simulink model "Udan_SOC"  (R2017b)
settings: Solver=FixedStepAuto  StartTime=0.0  StopTime=1000  FixedStep=0.1  RelTol=1e-3
values from neighbouring files (symbols this model uses):
  DenominatorOfIntegratorFactor = 100.0    [SOC_Stateflow.sldd]
  SOC_CalcSohLKT = 1.0    [SOC_Stateflow.sldd]
  SOC_CalcSOHTempLimit = 70.0    [SOC_Stateflow.sldd]
  SOC_CapPerCycle = 100.0    [SOC_Stateflow.sldd]
  SOC_CapTemp_HLimit = 200.0    [SOC_Stateflow.sldd]
  SOC_CapTemp_LLimit = 0.0    [SOC_Stateflow.sldd]
  Soc_ConfigInfo = 0    [SOC_Stateflow.sldd]
  SOC_DchgEndCalib = 0.0    [SOC_Stateflow.sldd]
  SOC_DiffVoltMin = 10.0    [SOC_Stateflow.sldd]
  SOC_DSOCJumpMax = 500.0    [SOC_Stateflow.sldd]
  SOC_EfficientHighLimit = 250.0    [SOC_Stateflow.sldd]
  SOC_EfficientLowLimit = 40.0    [SOC_Stateflow.sldd]
  SOC_EmptyAus = 0.0    [SOC_Stateflow.sldd]
  SOC_EnableOcv = 1.0    [SOC_Stateflow.sldd]
  SOC_END_CALIB_STATE : value not decoded    [SOC_Stateflow.sldd]
  SOC_HighRealSoc = 95.0    [SOC_Stateflow.sldd]
  SOC_LKTSohCycles = 0.0 1.0 10.0 20.0 30.0 40.0 50.0 60.0 70.0 80.0 90.0 100.0 110.0 120.0 130.0 140.0 150.0 160.0 170.0 180.0 190.0 200.0 210.0 220.0 230.0 240.0 250.0 260.0 270.0 280.0 290.0 300.0 310.0 320.0 330.0 340.0 350.0 360.0 370.0 380.0 390.0 400.0 410.0 420.0 430.0 440.0 450.0 460.0 470.0 480.0 490.0 500.0 510.0 520.0 530.0 540.0 550.0 560.0 570.0 580.0 590.0 600.0 610.0 620.0 630.0 640.0 650.0 660.0 670.0    [SOC_Stateflow.sldd]
  SOC_LKTSohTable = 1000.0 991.0 989.0 992.0 993.0 995.0 994.0 993.0 1000.0 997.0 1002.0 1000.0 992.0 1000.0 989.0 992.0 989.0 994.0 989.0 993.0 994.0 994.0 994.0 993.0 991.0 991.0 992.0 993.0 991.0 985.0 985.0 985.0 979.0 975.0 978.0 984.0 982.0 974.0 975.0 972.0 972.0 975.0 977.0 977.0 974.0 971.0 973.0 971.0 966.0 968.0 965.0 959.0 957.0 956.0 957.0 954.0 955.0 951.0 954.0 951.0 942.0 942.0 940.0 942.0 947.0 949.0    [SOC_Stateflow.sldd]
  SOC_LowRealSoc = 5.0    [SOC_Stateflow.sldd]
  SOC_NominalCap_AmS = 576000000.0    [SOC_Stateflow.sldd]
  SOC_NominalVol = 4000.0    [SOC_Stateflow.sldd]
  SOC_OCVTemp_HLimit = 106.0    [SOC_Stateflow.sldd]
  SOC_OCVTemp_LLimit = 29.0    [SOC_Stateflow.sldd]
  SOC_ShortCalibDSoc = 1.0    [SOC_Stateflow.sldd]
  SOC_SOCResolution = 10000.0    [SOC_Stateflow.sldd]
  SOC_SohCalcCapPercent = 8.0    [SOC_Stateflow.sldd]
  SOC_SohCalcHighLimit = 60.0    [SOC_Stateflow.sldd]
  SOC_SohCalcLowLimit = 10.0    [SOC_Stateflow.sldd]
  SOC_SohCalcMidLimit = 30.0    [SOC_Stateflow.sldd]
  SOC_SOHResolution = 1000.0    [SOC_Stateflow.sldd]
  SOC_State = <binary blob, 1163 chars, not shown>    [SOC_Stateflow.sldd]
  SOC_TempCap_CapBuffer : value not decoded    [SOC_Stateflow.sldd]
  SOC_TempCap_TempBuffer : value not decoded    [SOC_Stateflow.sldd]
  SocOcvCalib_ConfigInfo = 0.0    [SOC_Stateflow.sldd]
  SocOcvCalib_SocBuffer1 : value not decoded    [SOC_Stateflow.sldd]
  SocOcvCalib_TempBuffer : value not decoded    [SOC_Stateflow.sldd]
  SocOcvCalib_VoltageBuffer1 = 3300.0 3303.0 3305.0 3307.0 3310.0 3311.0 3313.0 3314.0 3316.0 3317.0 3319.0 3320.0 3322.0 3323.0 3325.0 3322.0 3323.0 3325.0 3310.0 3313.0 3315.0 3317.0 3320.0 3321.0 3323.0 3324.0 3326.0 3327.0 3329.0 3330.0 3332.0 3333.0 3335.0 3332.0 3333.0 3335.0 3320.0 3323.0 3325.0 3327.0 3330.0 3331.0 3333.0 3334.0 3336.0 3337.0 3339.0 3340.0 3342.0 3343.0 3345.0 3342.0 3343.0 3345.0 3330.0 3333.0 3335.0 3    [SOC_Stateflow.sldd]
  SOHCalibCycle = 10.0    [SOC_Stateflow.sldd]
undefined symbols (not defined in the file or in its folder): DatetimeM_GetReturnType, ParameterM_EeepParaIndexType, Soc_CumuLativeTypeType, SOC_EgthTempChgValue, Soc_EnergyBuffer, SOC_FithTempChgValue, SOC_FstSlowTempChgValue, SOC_FstTempChgValue, SOC_FthTempChgValue, SOC_MaxCap_AmS, SOC_SethTempChgValue, SOC_SixTempChgValue, SOC_SndSlowTempChgValue, SOC_SndTempChgValue, SOC_TrdSlowTempChgValue, SOC_TrdTempChgValue, SocDiagCalib_NoCalibReasonType
libraries: simulink x138, hdlsllib x24, dspindex x4
(part 2 of 10)

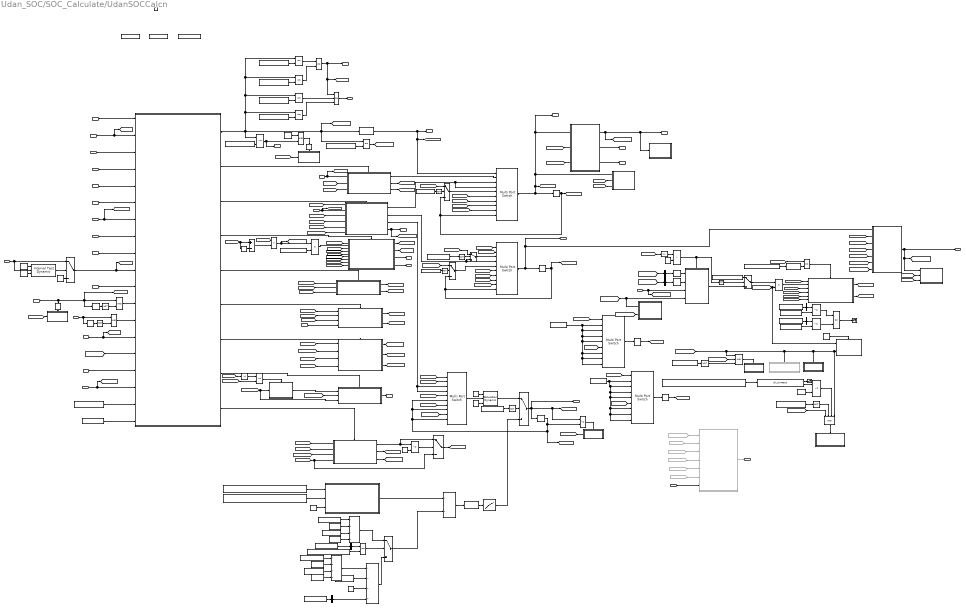
== system Udan_SOC/SOC_Calculate/UdanSOCCalcn ==
  note: 充电连接或者断开将未进行末端校正的累积安时数清0
  RtcTimeIsOk : Inport
  RtcTime : Inport  Port=2
  IsCharging : Inport  Port=3
  BmuStateIsOk : Inport  Port=4
  LongBatOffTimeOk : Inport  Port=5
  BatOffTimeOk : Inport  Port=6
  SohTimeOk : Inport  Port=7
  CalibCurrentMax : Inport  Port=8
  CalibCheckCycle : Inport  Port=9
  CalibWriteCycle : Inport  Port=10
  powerOnDelay : Inport  Port=11
  Current : Inport  Port=12
  LastOcvTime : Inport  Port=13
  FullChgFns : Inport  Port=14
  EmptyDchgFlag : Inport  Port=15
  EmptyValue : Inport  Port=16
  TimeStamps : Inport  Port=17
  CellLowTemp : Inport  Port=18
  UCell : Inport  Port=19
  SocCalibFlag : Inport  Port=20  OutDataTypeStr=uint8  PortDimensions=[1]
  BatHighTemp : Inport  Port=21
  Enable : EnablePort
  1-D Lookup Table : Lookup_n-D  NumberOfTableDimensions=1  BreakpointsForDimension1=SOC_LKTSohCycles  Table=SOC_LKTSohTable  ExtrapMethod=Clip  InternalRulePriority=Speed  OutDataTypeStr=uint16  RndMeth=Simplest
  Abs : Abs
  Abs1 : Abs
  Bus Selector : BusSelector  OutputSignals=soc
  Bus Selector1 : BusSelector  OutputSignals=soc
  Bus Selector2 : BusSelector  OutputSignals=DchgCumuInfo.resoltion
  Bus Selector4 : BusSelector  OutputSignals=DchgCumuInfo.type
  Bus Selector7 : BusSelector  OutputSignals=ChgCumuInfo.type
  Bus Selector8 : BusSelector  OutputSignals=DchgCumuInfo.type
  CalcChgSOH : Subsystem  TreatAsAtomicUnit=on
  CalcDchgSOH : Subsystem  TreatAsAtomicUnit=on
  CalcSocEffiient : Subsystem
  CalclnCore : Stateflow chart  TreatAsAtomicUnit=on
  CalcnLeftChargeTime : Subsystem  Commented=on
  CalcnSOC : Subsystem
  CalcnSOC1 : Subsystem
  CalibEmptySOC : Subsystem  TreatAsAtomicUnit=on
  CalibFullSOC : Subsystem  TreatAsAtomicUnit=on
  CapAdder1 : Subsystem
  CapAdder2 : Subsystem
  ClearLeftCapWOCalib : Subsystem  Commented=on
  ClearLeftCapWOCalib2 : Subsystem  TreatAsAtomicUnit=on
  ClearSOHCalcFlag : Subsystem  TreatAsAtomicUnit=on
  Constant : Constant  Value=0  OutDataTypeStr=uint8
  Constant1 : Constant  Value=DenominatorOfIntegratorFactor  OutDataTypeStr=uint16
  Constant10 : Constant  Value=600  OutDataTypeStr=uint16
  Constant11 : Constant  Value=0  OutDataTypeStr=uint32
  Constant12 : Constant  Value=0  OutDataTypeStr=int16
  Constant{13..14,25,27} (4 alike) : Constant  Value=Soc_ConfigInfo  OutDataTypeStr=Bus: Soc_ConfigInfoType
  Constant15 : Constant  Value=0  OutDataTypeStr=boolean
  Constant16 : Constant  Value=SOC_NominalCap_AmS
  Constant17 : Constant  Value=3600000  OutDataTypeStr=uint32
  Constant18 : Constant  Value=SOC_CalcSohLKT
  Constant19 : Constant  Value=SOC_CalcSohLKT
  Constant2 : Constant  Value=0
  Constant20 : Constant  Value=SOC_ShortCalibDSoc
  Constant21 : Constant  Value=SOC_CalcSohLKT
  Constant22 : Constant  Value=SOC_CapPerCycle  OutDataTypeStr=uint8
  Constant23 : Constant  Value=100  OutDataTypeStr=uint8
  Constant24 : Constant  OutDataTypeStr=boolean
  Constant26 : Constant  Value=10  OutDataTypeStr=uint8
  Constant28 : Constant  Value=SOC_NominalVol
  Constant29 : Constant  Value=SOC_NominalCap_AmS
  Constant3 : Constant  Value=65535  OutDataTypeStr=uint16
  Constant30 : Constant  Value=3600000  OutDataTypeStr=uint32
  Constant31 : Constant  Value=SOC_CapPerCycle  OutDataTypeStr=uint8
  Constant32 : Constant  Value=100  OutDataTypeStr=uint8
  Constant34 : Constant  Value=SOC_EnableOcv
  Constant4 : Constant  Value=SOC_EmptyAus
  Constant5 : Constant  Value=SOC_EmptyAus
  Constant6 : Constant  Value=20000  OutDataTypeStr=int16
  Constant7 : Constant  Value=-20000  OutDataTypeStr=int16
  Constant8 : Constant  Value=DenominatorOfIntegratorFactor  OutDataTypeStr=uint16
  Constant9 : Constant  Value=1100  OutDataTypeStr=uint16
  DLeftCap : MultiPortSwitch  DataPortOrder=Zero-based contiguous  Inputs=9  DataPortIndices={SOC_STATE_INIT,SOC_STATE_OCV,SOC_STATE_OCV_LONG,SOC_STATE_INTEGRATE,SOC_STATE_FULL}  OutDataTypeStr=uint32
  DLeftCap1 : MultiPortSwitch  DataPortOrder=Zero-based contiguous  Inputs=8  DataPortIndices={SOC_STATE_INIT,SOC_STATE_OCV,SOC_STATE_OCV_LONG,SOC_STATE_INTEGRATE,SOC_STATE_FULL}
  DLeftCap2 : MultiPortSwitch  DataPortOrder=Zero-based contiguous  Inputs=8  DataPortIndices={SOC_STATE_INIT,SOC_STATE_OCV,SOC_STATE_OCV_LONG,SOC_STATE_INTEGRATE,SOC_STATE_FULL}
  Data Store Memory1 : DataStoreMemory  DataStoreName=LargeCurrentFlag  ReadBeforeWriteMsg=warning  WriteAfterWriteMsg=warning  WriteAfterReadMsg=warning  ShowAdditionalParam=off  OutDataTypeStr=boolean
  Data Store Memory2 : DataStoreMemory  DataStoreName=FullFnshFlag  ReadBeforeWriteMsg=warning  WriteAfterWriteMsg=warning  WriteAfterReadMsg=warning  ShowAdditionalParam=off  OutDataTypeStr=boolean
  Data Store Memory4 : DataStoreMemory  DataStoreName=ChgClearWOCalibFlag  ReadBeforeWriteMsg=warning  WriteAfterWriteMsg=warning  WriteAfterReadMsg=warning  ShowAdditionalParam=off  OutDataTypeStr=boolean
  Data Store Read : DataStoreRead  DataStoreName=ChgClearWOCalibFlag
  Data Store Read1 : DataStoreRead  DataStoreName=LargeCurrentFlag
  Data Store Read2 : DataStoreRead  DataStoreName=FullFnshFlag
  Data Type Conversion : DataTypeConversion  OutDataTypeStr=uint8
  Data Type Conversion1 : DataTypeConversion  OutDataTypeStr=uint8
  Data Type Conversion2 : DataTypeConversion
  DchgPower1 : simulink/Sources/Enumerated Constant  OutDataTypeStr=Enum: ParameterM_EeepParaIndexType  Value=ParameterM_EeepParaIndexType.PARAMETERM_EEEP_CUMULATIVE_DCHG_CAP_L_INDEX  SampleTime=inf
      settings: SourceProductName=Simulink
  DchgPower2 : simulink/Sources/Enumerated Constant  OutDataTypeStr=Enum: ParameterM_EeepParaIndexType  Value=ParameterM_EeepParaIndexType.PARAMETERM_EEEP_SOH_Full_INDEX  SampleTime=inf
      settings: SourceProductName=Simulink
  DchgPower3 : simulink/Sources/Enumerated Constant  OutDataTypeStr=Enum: ParameterM_EeepParaIndexType  Value=ParameterM_EeepParaIndexType.PARAMETERM_EEEP_CUMULATIVE_DCHG_CAP_H_INDEX  SampleTime=inf
      settings: SourceProductName=Simulink
  Delay{,1..3,5..11} (11 alike) : Delay  DelayLength=1  InitialCondition=0
  Delay4 : Delay  InitialCondition=0
  Divide : Product  Inputs=*/*/  OutDataTypeStr=uint32
  Divide1 : Product  Inputs=*/  OutDataTypeStr=uint32  RndMeth=Round
  Divide3 : Product  Inputs=**  OutDataTypeStr=int32
  Divide4 : Product  Inputs=**  OutDataTypeStr=int32
  Divide6 : Product  Inputs=*/*/  OutDataTypeStr=uint32
  Divide7 : Product  Inputs=**//  OutDataTypeStr=uint32  RndMeth=Round
  Enabled Subsystem : Subsystem  TreatAsAtomicUnit=on
  Enumerated Constant : simulink/Sources/Enumerated Constant  OutDataTypeStr=Enum: SOC_State  Value=SOC_State.SOC_STATE_INTEGRATE  SampleTime=inf
      settings: SourceProductName=Simulink
  Enumerated Constant1 : simulink/Sources/Enumerated Constant  OutDataTypeStr=Enum: Soc_CumuLativeTypeType  Value=Soc_CumuLativeTypeType.Soc_CumuTypeNone  SampleTime=inf
      settings: SourceProductName=Simulink
  Enumerated Constant12 : simulink/Sources/Enumerated Constant  OutDataTypeStr=Enum: SOC_State  Value=SOC_State.SOC_STATE_INTEGRATE  SampleTime=inf
      settings: SourceProductName=Simulink
  Enumerated Constant2 : simulink/Sources/Enumerated Constant  OutDataTypeStr=Enum: Soc_CumuLativeTypeType  Value=Soc_CumuLativeTypeType.Soc_CumuTypeNone  SampleTime=inf
      settings: SourceProductName=Simulink
  Enumerated Constant3 : simulink/Sources/Enumerated Constant  OutDataTypeStr=Enum: SOC_State  Value=SOC_State.SOC_STATE_INIT  SampleTime=inf
      settings: SourceProductName=Simulink
  Enumerated Constant4 : simulink/Sources/Enumerated Constant  OutDataTypeStr=Enum: SOC_State  Value=SOC_State.SOC_STATE_FULL  SampleTime=inf
      settings: SourceProductName=Simulink
  Enumerated Constant5 : simulink/Sources/Enumerated Constant  OutDataTypeStr=Enum: SOC_State  Value=SOC_State.SOC_STATE_EMPTY  SampleTime=inf
      settings: SourceProductName=Simulink
  Enumerated Constant6 : simulink/Sources/Enumerated Constant  OutDataTypeStr=Enum: SOC_State  Value=SOC_State.SOC_STATE_OCV_LONG  SampleTime=inf
      settings: SourceProductName=Simulink
  Enumerated Constant7 : simulink/Sources/Enumerated Constant  OutDataTypeStr=Enum: SOC_State  Value=SOC_State.SOC_STATE_OCV  SampleTime=inf
      settings: SourceProductName=Simulink
  Enumerated Constant8 : simulink/Sources/Enumerated Constant  OutDataTypeStr=Enum: Soc_CumuLativeTypeType  Value=Soc_CumuLativeTypeType.Soc_CumuTypeCap  SampleTime=inf
      settings: SourceProductName=Simulink
  From74 : From  Commented=on  GotoTag=LastDCapWODelay
  From75 : From  Commented=on  GotoTag=CellTemp
  From77 : From  Commented=on  GotoTag=CurrentSOH
  From78 : From  Commented=on  GotoTag=IsCharging
  From84 : From  Commented=on  GotoTag=TimeStamps
  From92 : From  Commented=on  GotoTag=Current
  Function-Call Subsystem : Subsystem  TreatAsAtomicUnit=on
  Function-Call Subsystem4 : Subsystem  TreatAsAtomicUnit=on
  Interval Test Dynamic : simulink/Logic and Bit Operations/Interval Test Dynamic  IntervalClosedRight=on  IntervalClosedLeft=on  OutDataTypeStr=boolean
      settings: SourceProductName=Simulink  SourceProductBaseCode=SL
  LKTSOC : Subsystem  TreatAsAtomicUnit=on
  LeftCap : MultiPortSwitch  DataPortOrder=Zero-based contiguous  Inputs=9  DataPortIndices={SOC_STATE_INIT,SOC_STATE_OCV,SOC_STATE_OCV_LONG,SOC_STATE_INTEGRATE,SOC_STATE_FULL}  OutDataTypeStr=uint32
  Logical Operator : Logic  Inputs=4  AllPortsSameDT=off  OutDataTypeStr=boolean
  Logical Operator{1,3,8,12..16} (8 alike) : Logic  Operator=NOT  AllPortsSameDT=off  OutDataTypeStr=boolean
  Logical Operator10 : Logic  Operator=OR  AllPortsSameDT=off  OutDataTypeStr=boolean
  Logical Operator11 : Logic  AllPortsSameDT=off  OutDataTypeStr=boolean
  Logical Operator2 : Logic  AllPortsSameDT=off  OutDataTypeStr=boolean
  Logical Operator4 : Logic  Inputs=3  AllPortsSameDT=off  OutDataTypeStr=boolean
  Logical Operator5 : Logic  Operator=OR  AllPortsSameDT=off  OutDataTypeStr=boolean
  Logical Operator6 : Logic  Operator=NOT  Inputs=3  AllPortsSameDT=off  OutDataTypeStr=boolean
  Logical Operator7 : Logic  Operator=OR  Inputs=3  AllPortsSameDT=off  OutDataTypeStr=boolean
  Logical Operator9 : Logic  AllPortsSameDT=off  OutDataTypeStr=boolean
  Multiport Switch1 : MultiPortSwitch  DataPortOrder=Zero-based contiguous  Inputs=9  DataPortIndices={SOC_STATE_INIT,SOC_STATE_OCV,SOC_STATE_OCV_LONG,SOC_STATE_INTEGRATE,SOC_STATE_FULL}
  Product : Product  OutDataTypeStr=int32
  Relational Operator{,7..8,10..12,15} (7 alike) : RelationalOperator  Operator===  OutDataTypeStr=boolean  RndMeth=Simplest
  Relational Operator{1..6} (6 alike) : RelationalOperator  Operator=~=  OutDataTypeStr=boolean  RndMeth=Simplest
  Relational Operator13 : RelationalOperator  OutDataTypeStr=boolean  RndMeth=Simplest
  Relational Operator9 : RelationalOperator  Operator=>  OutDataTypeStr=boolean  RndMeth=Simplest
  S-Function2 : S-Function  FunctionName=sfn_NVMRead  SFunctionDeploymentMode=off  EnableBusSupport=off
  Saturation Dynamic : simulink/Discontinuities/Saturation Dynamic  OutMin=[]  OutMax=[]  OutDataTypeStr=Inherit: Same as second input  OutDataType=fixdt(1, 16)  OutScaling=2^-10  DoSatur=off
  SetSOHCalcFlag : Subsystem  TreatAsAtomicUnit=on
  SetSOHCalcFlagFullChg : Subsystem  TreatAsAtomicUnit=on
  StoreCulumutiveAh : Subsystem  TreatAsAtomicUnit=on
  StoreDSOC : Subsystem
  StoreLeftCap : Subsystem
  StoreSOC : Subsystem  TreatAsAtomicUnit=on
  StoreTSOC : Subsystem
  Subsystem1 : Subsystem  mask(ReadEeep_uint32){}
  Subtract : Sum  Inputs=+-  OutDataTypeStr=int32
  Switch{,3..7} (6 alike) : Switch  Criteria=u2 > Threshold
  Switch1 : Switch  Criteria=u2 > Threshold  OutDataTypeStr=int16
  Switch2 : Switch  Criteria=u2 > Threshold  OutDataTypeStr=uint16
  Terminator : Terminator
  Terminator1 : Terminator
  WriteOCVTime : Subsystem  TreatAsAtomicUnit=on
  WriteSOH : Subsystem  TreatAsAtomicUnit=on
  SOC_State : Outport
  SocParam : Outport  Port=2
  SocDParam : Outport  Port=3
  SOC_LeftCap : Outport  Port=4
  SOC_DLeftCap : Outport  Port=5
  SOC_SohOut : Outport  Port=6
  SOC_SocInitFns : Outport  Port=7
  SOC_ClearBufferCmd : Outport  Port=8
  SOC_LeftEnergy : Outport  Port=9
  SOC_RealSoc : Outport  Port=10
  LeftCahrgeTime : Outport  Port=11
  CulumChargeAh : Outport  Port=12
  SOC_OcvCmd : Outport  Port=13
  CulumDchargeAh : Outport  Port=14
  SOC_RTCTime : Outport  Port=15
  LookUpLeftCap : Outport  Port=16
  wires:
  CalcChgSOH/2(NewCap) -> [FullCalibSOHCap]
  [ChgSOH] -> Multiport Switch1/5
  [LastCap] -> CalcChgSOH/1(Capacity)
  LeftCap/1 -> [NowCap], SOC_LeftCap/1, CalcnSOC/1(LeftCap), StoreLeftCap/1(LastCap), Delay/1
  [LastCap] -> SetSOHCalcFlagFullChg/1(LastCap)
  DLeftCap/1 -> Delay3/1, CalcnSOC1/1(LeftCap), SOC_DLeftCap/1  "SOC_DLeftCap"
  [Current] -> CalcnSOC1/2(Current)
  [CurrentSOH] -> CalcnSOC1/5(SohOut)
  [CellTemp] -> CalcnSOC1/4(AverageTemp)
  [FullChgFns] -> CalcnSOC1/3(FullCharge)
  [TempCapResolution] -> CalcnSOC1/6(TempCapResolution)
  CapAdder2/1(NewCap) -> [IntergrateDCap]
  Divide4/1 -> CapAdder1/2(AmpereMicrosec)
  Constant1/1 -> Divide4/2
  [TimeStamps] -> Delay1/1, Subtract/1
  CalcnSOC1/1(SOCParam) -> [DSocParam], StoreDSOC/1(LastCap), SocDParam/1
  CalcnSOC/1(SOCParam) -> [SocParam], StoreTSOC/1(LastCap), SocParam/1
  [CurrentSOH] -> CalcnSOC/3(SohOut)
  [CellTemp] -> CalcnSOC/2(AverageTemp)
  [EmptyCap] -> LeftCap/8
  [LastCap] -> CalibEmptySOC/1(Capacity)
  [LastSOH] -> CalibEmptySOC/2(SOH)
  CalclnCore/6(CalibEmptySOC()) -> CalibEmptySOC/Trigger
  Logical Operator11/1 -> CalclnCore/13(EmptyDchgFlag)
  FullChgFns/1 -> Logical Operator2/1, [FullChgFns], Delay10/1, Delay4/1
  LastOcvTime/1 -> CalclnCore/11(LastTime)
  RtcTime/1 -> CalclnCore/2(NowTime), [RtcTime]
  CalibWriteCycle/1 -> CalclnCore/9(CalibCycle)
  CalibCheckCycle/1 -> CalclnCore/8(checkCycle)
  Switch1/1 -> CalclnCore/10(Current), [Current]
  CalibCurrentMax/1 -> CalclnCore/7(CurrentMax), [CalibCurrentMax]
  SohTimeOk/1 -> CalclnCore/6(SohTimeDiffOk)
  BatOffTimeOk/1 -> CalclnCore/5(BatOffTimeOk)
  LongBatOffTimeOk/1 -> CalclnCore/4(LongBatOffTimeOk)
  BmuStateIsOk/1 -> CalclnCore/3(BmuStateIsOk)
  RtcTimeIsOk/1 -> CalclnCore/1(RtcTimeIsOk)
  Bus Selector7/1 -> Relational Operator4/1  "<type>"
  Constant13/1 -> Bus Selector7/1
  IsCharging/1 -> CalcSocEffiient/3(IsCharging), [IsCharging]
  [IsCharging] -> Logical Operator4/1, Function-Call Subsystem/Trigger, Logical Operator/4, StoreCulumutiveAh/2(IsCharging), ClearLeftCapWOCalib/Trigger
  [AmpereMicrosec] -> StoreCulumutiveAh/1(Cap_TenthAmS), Product/2
  Relational Operator5/1 -> Logical Operator5/2
  Logical Operator5/1 -> Terminator1/1
  Enumerated Constant1/1 -> Relational Operator4/2
  Constant14/1 -> Bus Selector8/1
  Bus Selector8/1 -> Relational Operator5/1  "<type>"
  Enumerated Constant2/1 -> Relational Operator5/2
  Relational Operator4/1 -> Logical Operator5/1
  Data Type Conversion1/1 -> Relational Operator/2
  Delay3/1 -> DLeftCap/10, Switch6/3, [LastDCap]
  [SocParam] -> Bus Selector/1
  [AmpereMicrosec] -> StoreSOC/1(CurrentAmS), CalcSocEffiient/4(Current)
  Relational Operator/1 -> CapAdder2/Enable
  Enumerated Constant/1 -> Data Type Conversion1/1
  [State] -> Relational Operator/1
  [LastDCap] -> CapAdder2/1(Capacity)
  Product/1 -> CapAdder2/2(AmpereMicrosec)
  Switch2/1 -> Product/1
  [FullDCap] -> DLeftCap/7
  [IntergrateDCap] -> DLeftCap/6
  [EEEPDLeftCap] -> DLeftCap/2
  [State] -> DLeftCap/1
  [FullCap] -> LeftCap/7
  [IntergrateCap] -> LeftCap/6
  Delay/1 -> Switch5/3, LeftCap/10, [LastCap]
  Function-Call Subsystem4/1(EEEPLeftCap) -> LeftCap/2
  [State] -> Multiport Switch1/1
  Delay2/1 -> Relational Operator1/2, [LastSOH], Multiport Switch1/10, Multiport Switch1/6, Multiport Switch1/8
  Relational Operator1/1 -> WriteSOH/Enable
  [CurrentSOH] -> WriteSOH/1(SOH)
  [InitSOH] -> Multiport Switch1/2
  Function-Call Subsystem4/2(EEEPSOH) -> [InitSOH]
  CapAdder1/1(NewCap) -> [IntergrateCap]
  CalibFullSOC/1(NewCap) -> [FullCap]
  [ChgSOH] -> Multiport Switch1/7
  [LastSOH] -> LKTSOC/3(SOH)
  [LastSOH] -> CalibFullSOC/2(SOH)
  [LastSOH] -> CalcChgSOH/4(SOHIn), Switch/3
  [LastCap] -> CalibFullSOC/1(Capacity)
  [LastCap] -> CapAdder1/1(Capacity)
  CalclnCore/4(SOCIntegrate()) -> CapAdder1/Trigger
  CalclnCore/3(LookUpOcvTable()) -> LKTSOC/Trigger
  CalcChgSOH/1(SohOut) -> Relational Operator6/1, Switch/1
  LKTSOC/3(SohOut) -> Multiport Switch1/3, Multiport Switch1/4
  CalclnCore/9(CalcChgSOH()) -> CalcChgSOH/Trigger
  [Current] -> Divide3/1
  Divide3/1 -> [AmpereMicrosec], Divide4/1  "I*T"
  CalclnCore/2(InitSOC()) -> Function-Call Subsystem4/Trigger
  CalclnCore/5(CalibFullSOC()) -> CalibFullSOC/Trigger
  CellLowTemp/1 -> [CellTemp], Function-Call Subsystem4/1(CellLowTemp)
  UCell/1 -> LKTSOC/2(UCell), [CellVol]
  CalclnCore/8(WriteOCVTime()) -> WriteOCVTime/Trigger
  Delay1/1 -> Subtract/2
  Subtract/1 -> Divide3/2
  Logical Operator9/1 -> Delay6/1
  Constant15/1 -> Logical Operator9/1
  Delay6/1 -> SetSOHCalcFlag/Trigger
  [LastCap] -> SetSOHCalcFlag/1(SocParam)
  Enumerated Constant3/1 -> Relational Operator3/2
  Relational Operator3/1 -> SOC_SocInitFns/1, Logical Operator9/2
  DchgPower2/1 -> S-Function2/1
  S-Function2/2 -> Relational Operator2/1
  Constant3/1 -> Relational Operator2/2
  Logical Operator/1 -> ClearSOHCalcFlag/Enable
  Relational Operator2/1 -> Logical Operator/3
  S-Function2/1 -> Terminator/1
  SocCalibFlag/1 -> CalclnCore/14(SocCalibFlag), [SocCalibFlag]
  Data Type Conversion/1 -> LeftCap/1, [State], SOC_State/1
  Constant/1 -> Relational Operator6/2
  Relational Operator6/1 -> Switch/2
  Switch/1 -> [ChgSOH]
  [IsCharging] -> CalclnCore/15(IsCharging)
  Data Store Read2/1 -> Logical Operator1/1
  Logical Operator1/1 -> Logical Operator/2
  Delay4/1 -> SetSOHCalcFlagFullChg/Trigger
  [CellTemp] -> CapAdder1/4(CellLowTemp)
  [LastSOH] -> CapAdder1/6(SOH)
  Function-Call Subsystem4/3(EEEPDLeftCap) -> [EEEPDLeftCap]
  [EmptyDCap] -> DLeftCap/8
  LKTSOC/1(LeftCap) -> LeftCap/3, LeftCap/4
  [CellTemp] -> LKTSOC/1(CellLowTemp)
  [IsCharging] -> CapAdder1/7(IsCharging)
  [LastCap] -> LKTSOC/4(Capacity)
  [SocCalibFlag] -> Function-Call Subsystem4/2(SocCalibFlag)
  [State] -> DLeftCap1/1
  Constant4/1 -> DLeftCap1/7, DLeftCap1/9, DLeftCap1/8, DLeftCap1/5, DLeftCap1/4, DLeftCap1/3, DLeftCap1/2  "AuS"
  DLeftCap1/1 -> Delay5/1
  CapAdder1/2(LeftCapAusOut) -> [LeftCapAusOut]
  [LeftCapAusOut] -> DLeftCap1/6
  [DLeftCapAusIn] -> CapAdder2/3(LeftCapAusIn)
  [State] -> DLeftCap2/1
  Constant5/1 -> DLeftCap2/8, DLeftCap2/9, DLeftCap2/7, DLeftCap2/5, DLeftCap2/4, DLeftCap2/3, DLeftCap2/2
  CapAdder2/2(LeftCapAusOut) -> [DLeftCapAusOut]
  [DLeftCapAusOut] -> DLeftCap2/6
  DLeftCap2/1 -> Delay7/1
  Delay5/1 -> [LeftCapAusIn]
  Delay7/1 -> [DLeftCapAusIn]
  [IsCharging] -> StoreSOC/2(IsCharging)
  [FullCalibSOHCap] -> Switch5/1
  [NowCap] -> CapAdder2/4(NowCap)
  [SocCalibFlag] -> StoreLeftCap/3(SocCalibFlag)
  [SocCalibFlag] -> StoreDSOC/2(SocCalibFlag)
  Current/1 -> Interval Test Dynamic/2, Switch1/1
  Interval Test Dynamic/1 -> Switch1/2
  Constant6/1 -> Interval Test Dynamic/1
  Constant7/1 -> Interval Test Dynamic/3
  Constant12/1 -> Switch1/3
  LKTSOC/2(DLeftCap) -> Switch4/3, DLeftCap/4
  [DSocParam] -> Bus Selector1/1
  Bus Selector/1 -> Delay8/1  "<soc>"
  Bus Selector1/1 -> Delay9/1  "<soc>"
  Delay8/1 -> CalcSocEffiient/1(SOC)
  Delay9/1 -> CalcSocEffiient/2(DSOC)
  CalibFullSOC/2(NewDCap) -> [FullDCap]
  [LastDCap] -> CalcChgSOH/2(DCapacity)
  CalcChgSOH/3(DNewCap) -> [FullCalibSOHDCap]
  CalibEmptySOC/2(NewDCap) -> [EmptyDCap]
  CalibEmptySOC/1(NewCap) -> [EmptyCap]
  [CellTemp] -> CalibEmptySOC/3(AverageTemp)
  Relational Operator15/1 -> [State_Integrat]
  Enumerated Constant12/1 -> Relational Operator15/2
  Logical Operator4/1 -> ClearLeftCapWOCalib2/Enable
  [State_Integrat] -> Logical Operator4/2
  Logical Operator6/1 -> Logical Operator4/3
  Data Store Read/1 -> Logical Operator6/1
  [State_Integrat] -> Logical Operator/1
  Logical Operator2/1 -> CalclnCore/12(FullChgFns)
  [IsCharging] -> CalcnSOC1/7(IsCharging)
  Delay10/1 -> Logical Operator3/1
  Logical Operator3/1 -> Logical Operator2/2
  Enumerated Constant4/1 -> Relational Operator7/2
  Enumerated Constant5/1 -> Relational Operator8/2
  Relational Operator8/1 -> Logical Operator7/2
  Relational Operator7/1 -> Logical Operator7/3
  Logical Operator7/1 -> SOC_ClearBufferCmd/1
  [State_LongCailb] -> LKTSOC/6(Soc_State)
  [Current] -> Abs/1
  Abs/1 -> Relational Operator9/1
  Constant2/1 -> Relational Operator9/2
  Relational Operator9/1 -> CalcSocEffiient/Enable, Logical Operator8/1
  Logical Operator8/1 -> Switch2/2
  CalcSocEffiient/1(OcvFactor) -> Switch2/3
  Constant8/1 -> Switch2/1
  CalcnSOC/2(SOC_LeftEnergy) -> SOC_LeftEnergy/1
  CalcnSOC/3(SOC_RealSoc) -> SOC_RealSoc/1
  CalcnLeftChargeTime/1(LeftCahrgeTime) -> LeftCahrgeTime/1
  From78/1 -> CalcnLeftChargeTime/1(ChargeType)
  From92/1 -> CalcnLeftChargeTime/2(Current)
  From84/1 -> CalcnLeftChargeTime/3(TimeStamps)
  From74/1 -> CalcnLeftChargeTime/4(DleftCap)
  From75/1 -> CalcnLeftChargeTime/5(CellTemp)
  CapAdder1/3(CulumChargeAh) -> CulumChargeAh/1
  Relational Operator11/1 -> Logical Operator10/2
  Logical Operator10/1 -> SOC_OcvCmd/1, [OcvCmd], Logical Operator7/1
  Relational Operator10/1 -> Logical Operator10/1
  Enumerated Constant6/1 -> Relational Operator11/2
  Enumerated Constant7/1 -> Relational Operator10/2
  Constant9/1 -> Saturation Dynamic/1
  Multiport Switch1/1 -> Saturation Dynamic/2  "SOC_SohOut"
  Constant10/1 -> Saturation Dynamic/3
  Logical Operator12/1 -> Logical Operator11/2
  EmptyDchgFlag/1 -> Delay11/1, Logical Operator11/1
  Delay11/1 -> Logical Operator12/1
  [LastSOH] -> CapAdder2/5(SOH)
  From77/1 -> CalcnLeftChargeTime/6(SOH)
  BatHighTemp/1 -> CalcnLeftChargeTime/7(BatHighTemp)
  CapAdder1/4(CulumDchargeAh) -> CulumDchargeAh/1
  [CellVol] -> Function-Call Subsystem4/3(UCell)
  CalcDchgSOH/2(NewCap) -> [DchgSOHCap]
  [LastCap] -> CalcDchgSOH/3(Capacity)
  CalcDchgSOH/3(DNewCap) -> [DchgSOHDCap]
  CalcDchgSOH/1(SohOut) -> [DchgSOH]
  CalclnCore/7(CalcDchgSOH()) -> CalcDchgSOH/Trigger
  [LookUpLeftCap] -> CalcDchgSOH/2(SOC_LeftCap2)
  [LastDCap] -> CalcDchgSOH/4(DCapacity)
  [LastSOH] -> CalcDchgSOH/1(SOHIn)  "LstSOH"
  LKTSOC/4(LookUpLeftCap) -> LookUpLeftCap/1, [LookUpLeftCap]
  [DchgSOHCap] -> LeftCap/9
  [DchgSOHDCap] -> DLeftCap/9
  [DchgSOH] -> Multiport Switch1/9
  [SocCalibFlag] -> CapAdder1/9(SocCalibFlag)
  [SocCalibFlag] -> CapAdder2/6(SocCalibFlag)
  [CellTemp] -> CalibFullSOC/3(BatTemp)
  DchgPower1/1 -> Subsystem1/2(LowIndex)
  DchgPower3/1 -> Subsystem1/1(HighIndex)
  Constant11/1 -> Subsystem1/3(DefaultValue)
  Constant17/1 -> Divide/2
  Subsystem1/1(EeepRead32) -> Divide1/1
  Divide1/1 -> Data Type Conversion2/1
  Saturation Dynamic/1 -> Switch3/1  "SOC_SohOut"
  Data Type Conversion2/1 -> 1-D Lookup Table/1
  [LastDCap] -> Switch4/1
  [Current] -> CapAdder1/3(Current100mA)
  [LeftCapAusIn] -> CapAdder1/8(LeftCapAusIn)
  [CellVol] -> CapAdder1/5(UCell)
  Logical Operator13/1 -> Switch3/2
  1-D Lookup Table/1 -> Switch3/3  "SOC_SohOut"
  Switch3/1 -> SOC_SohOut/1, Delay2/1, Relational Operator1/1, [CurrentSOH]
  Logical Operator14/1 -> Switch4/2
  Switch4/1 -> DLeftCap/3
  Constant19/1 -> Logical Operator13/1
  Constant20/1 -> Logical Operator14/1
  Constant16/1 -> Divide/1
  Constant18/1 -> Logical Operator15/1
  Logical Operator15/1 -> Switch5/2
  Switch5/1 -> LeftCap/5
  Logical Operator16/1 -> Switch6/2
  Constant21/1 -> Logical Operator16/1
  [FullCalibSOHDCap] -> Switch6/1
  Switch6/1 -> DLeftCap/5
  Constant22/1 -> Divide/3
  Constant23/1 -> Divide/4
  Constant24/1 -> StoreCulumutiveAh/Enable
  Enumerated Constant8/1 -> Relational Operator12/2
  Bus Selector4/1 -> Relational Operator12/1  "<type>"
  Constant25/1 -> Bus Selector4/1
  Relational Operator12/1 -> Switch7/2
  Bus Selector2/1 -> Divide7/4  "<resoltion>"
  Constant27/1 -> Bus Selector2/1
  Constant28/1 -> Divide7/2
  Divide/1 -> Switch7/1
  Constant26/1 -> Divide7/3
  Switch7/1 -> Divide1/2
  Constant32/1 -> Divide6/4
  Constant31/1 -> Divide6/3
  Constant29/1 -> Divide6/1
  Constant30/1 -> Divide6/2
  Divide6/1 -> Divide7/1
  Divide7/1 -> Switch7/3
  powerOnDelay/1 -> CalclnCore/16(powerOnDelay)
  TimeStamps/1 -> [TimeStamps], CalclnCore/17(OSTime)
  [Current] -> Abs1/1
  [CalibCurrentMax] -> Relational Operator13/2
  Abs1/1 -> Relational Operator13/1
  [RtcTime] -> WriteOCVTime/3(RtcTime), Enabled Subsystem/1(RtcTimeIn)
  [LookUpLeftCap] -> CalcChgSOH/3(LookUpLeftCap)
  CalclnCore/1(SOC_State) -> Relational Operator10/1, Relational Operator11/1, Relational Operator8/1, Relational Operator7/1, Relational Operator3/1, [State_LongCailb], Data Type Conversion/1, Relational Operator15/1
  Relational Operator13/1 -> Enabled Subsystem/Enable
  [State_LongCailb] -> WriteOCVTime/2(OCVCmd)
  Enabled Subsystem/1(RtcTimeOut) -> WriteOCVTime/1(RTCTimeOut)
  Data Store Read1/1 -> CalclnCore/18(largeCurrentFlag)
  WriteOCVTime/1(SOC_RTCTime) -> SOC_RTCTime/1
  [OcvCmd] -> StoreLeftCap/2(OcvCmd)
  [OcvCmd] -> StoreDSOC/3(OcvCmd)
  Constant34/1 -> CalclnCore/19(EnableOcv)
  [LastDCap] -> LKTSOC/5(DCapacity)
  EmptyValue/1 -> CalibEmptySOC/4(EmptyValue)

== system Udan_SOC/SOC_Calculate/Subsystem1/Subsystem ==
  HighIndex : Inport
  LowIndex : Inport  Port=2
  Enable : EnablePort
  Add : Sum
  Bit Rotate : hdlsllib/Logic and Bit Operations/Bit Rotate  mode=Rotate Left  N=16
      settings: SourceProductName=HDL Coder  SourceProductBaseCode=HD
  Data Type Conversion : DataTypeConversion  OutDataTypeStr=uint32
  soc : Outport
  wires:
  LowIndex/1 -> Add/2
  Bit Rotate/1 -> Add/1
  Data Type Conversion/1 -> Bit Rotate/1
  HighIndex/1 -> Data Type Conversion/1
  Add/1 -> soc/1  "soc"

== system Udan_SOC/SOC_Calculate/UdanSOCCalcn/CalcChgSOH ==
  Capacity : Inport
  DCapacity : Inport  Port=2
  LookUpLeftCap : Inport  Port=3
  SOHIn : Inport  Port=4
  Trigger : TriggerPort  TriggerType=function-call  VariantControl=Variant  PortDimensions=1
  Constant : Constant  Value=10  OutDataTypeStr=uint8
  Constant1 : Constant  Value=SOC_SohCalcCapPercent  OutDataTypeStr=uint8
  Constant15 : Constant  Value=SOC_SOHResolution  OutDataTypeStr=uint16
  Constant2 : Constant  Value=0  OutDataTypeStr=uint32
  Constant31 : Constant  Value=SOC_NominalCap_AmS
  DchgPower2 : simulink/Sources/Enumerated Constant  OutDataTypeStr=Enum: ParameterM_EeepParaIndexType  Value=ParameterM_EeepParaIndexType.PARAMETERM_EEEP_LEFTCAP_WOCALIB_H_INDEX  SampleTime=inf
      settings: SourceProductName=Simulink
  DchgPower4 : simulink/Sources/Enumerated Constant  OutDataTypeStr=Enum: ParameterM_EeepParaIndexType  Value=ParameterM_EeepParaIndexType.PARAMETERM_EEEP_LEFTCAP_WOCALIB_L_INDEX  SampleTime=inf
      settings: SourceProductName=Simulink
  Divide{,1..2,5} (4 alike) : Product  Inputs=*/*  OutDataTypeStr=uint32
  Logical Operator1 : Logic  Operator=NOT  AllPortsSameDT=off  OutDataTypeStr=boolean
  Relational Operator : RelationalOperator  Operator=<  OutDataTypeStr=boolean  RndMeth=Simplest
  Subsystem : Subsystem
  Subsystem1 : Subsystem  mask(ReadEeep_uint32){}
  Switch : Switch  Criteria=u2 > Threshold
  SohOut : Outport
  NewCap : Outport  Port=2
  DNewCap : Outport  Port=3
  wires:
  Capacity/1 -> Divide1/1
  Divide1/1 -> NewCap/1  "AmS"
  [SOHIn] -> Divide1/2
  Subsystem/1(SohOut) -> Switch/3
  Logical Operator1/1 -> Switch/2
  [SOHIn] -> Switch/1
  Relational Operator/1 -> Subsystem/Enable, Logical Operator1/1  "ChgSOHCalcFlag"
  Divide/1 -> Relational Operator/1
  Constant/1 -> Divide/2
  SOHIn/1 -> [SOHIn], Subsystem/4(SOHIn)
  Divide5/1 -> Divide/1, Subsystem/2(TotalCap)
  DchgPower2/1 -> Subsystem1/1(HighIndex)
  DchgPower4/1 -> Subsystem1/2(LowIndex)
  Constant2/1 -> Subsystem1/3(DefaultValue)
  Subsystem1/1(EeepRead32) -> Subsystem/1(SOC_LeftCap), Relational Operator/2  "LeftCapWOCalib"
  Switch/1 -> SohOut/1, Divide2/3, Divide1/3
  [SOHIn] -> Divide2/2
  DCapacity/1 -> Divide2/1
  Divide2/1 -> DNewCap/1
  Constant1/1 -> Divide/3
  Constant15/1 -> Divide5/2
  Constant31/1 -> Divide5/1
  [SOHIn] -> Divide5/3
  LookUpLeftCap/1 -> Subsystem/3(LookUpLeftCap)

== system Udan_SOC/SOC_Calculate/UdanSOCCalcn/CalcDchgSOH ==
  SOHIn : Inport
  SOC_LeftCap2 : Inport  Port=2
  Capacity : Inport  Port=3
  DCapacity : Inport  Port=4
  function : TriggerPort  TriggerType=function-call  VariantControl=Variant
  Constant : Constant  Value=10  OutDataTypeStr=uint8
  Constant1 : Constant  Value=SOC_SOHResolution  OutDataTypeStr=uint16
  Constant2 : Constant  Value=0  OutDataTypeStr=uint32
  Constant3 : Constant  Value=SOC_SohCalcCapPercent  OutDataTypeStr=uint8
  Constant31 : Constant  Value=SOC_NominalCap_AmS
  Constant7 : Constant  Value=65535  OutDataTypeStr=uint16
  DchgPower1 : simulink/Sources/Enumerated Constant  OutDataTypeStr=Enum: ParameterM_EeepParaIndexType  Value=ParameterM_EeepParaIndexType.PARAMETERM_EEEP_SOH_Full_INDEX  SampleTime=inf
      settings: SourceProductName=Simulink
  DchgPower2 : simulink/Sources/Enumerated Constant  OutDataTypeStr=Enum: ParameterM_EeepParaIndexType  Value=ParameterM_EeepParaIndexType.PARAMETERM_EEEP_LEFTCAP_WOCALIB_H_INDEX  SampleTime=inf
      settings: SourceProductName=Simulink
  DchgPower4 : simulink/Sources/Enumerated Constant  OutDataTypeStr=Enum: ParameterM_EeepParaIndexType  Value=ParameterM_EeepParaIndexType.PARAMETERM_EEEP_LEFTCAP_WOCALIB_L_INDEX  SampleTime=inf
      settings: SourceProductName=Simulink
  Divide{,1..2,6} (4 alike) : Product  Inputs=*/*  OutDataTypeStr=uint32
  Logical Operator : Logic  AllPortsSameDT=off  OutDataTypeStr=boolean
  Logical Operator1 : Logic  Operator=NOT  AllPortsSameDT=off  OutDataTypeStr=boolean
  Relational Operator2 : RelationalOperator  Operator=<  OutDataTypeStr=boolean  RndMeth=Simplest
  Relational Operator3 : RelationalOperator  Operator=~=  OutDataTypeStr=boolean  RndMeth=Simplest
  S-Function1 : S-Function  FunctionName=sfn_NVMRead  SFunctionDeploymentMode=off  EnableBusSupport=off
  Subsystem : Subsystem
  Subsystem1 : Subsystem  mask(ReadEeep_uint32){}
  Switch : Switch  Criteria=u2 > Threshold
  Terminator1 : Terminator
  SohOut : Outport
  NewCap : Outport  Port=2
  DNewCap : Outport  Port=3
  wires:
  Divide/1 -> NewCap/1
  Capacity/1 -> Divide/1
  [SOHIn] -> Divide/2
  Subsystem/1(SohOut) -> Switch/3
  [SOHIn] -> Switch/1  "DCHSOHIN"
  Logical Operator1/1 -> Switch/2
  SOC_LeftCap2/1 -> Subsystem/2(SOC_LeftCap2)
  Logical Operator/1 -> Subsystem/Enable, Logical Operator1/1  "enablefalg"
  Subsystem1/1(EeepRead32) -> [WOCalibAh], Relational Operator2/2  "wocalib"
  Relational Operator2/1 -> Logical Operator/1  "enable2"
  Constant31/1 -> Divide1/1
  SOHIn/1 -> Divide1/3, Subsystem/3(SOHIn), [SOHIn]
  Divide6/1 -> Relational Operator2/1  "calcthr"
  Constant1/1 -> Divide1/2
  DchgPower2/1 -> Subsystem1/1(HighIndex)
  DchgPower4/1 -> Subsystem1/2(LowIndex)
  S-Function1/2 -> Subsystem/1(SOC_LeftCap0), Relational Operator3/1
  DchgPower1/1 -> S-Function1/1
  Constant7/1 -> Relational Operator3/2
  Relational Operator3/1 -> Logical Operator/2  "enable1"
  S-Function1/1 -> Terminator1/1
  [WOCalibAh] -> Subsystem/4(WOCalibAh)
  Constant2/1 -> Subsystem1/3(DefaultValue)
  Divide1/1 -> Divide6/1
  Constant/1 -> Divide6/2
  Constant3/1 -> Divide6/3
  [SOHIn] -> Divide2/2
  Divide2/1 -> DNewCap/1
  Switch/1 -> SohOut/1, Divide2/3, Divide/3  "DCHSOHOUt"
  DCapacity/1 -> Divide2/1

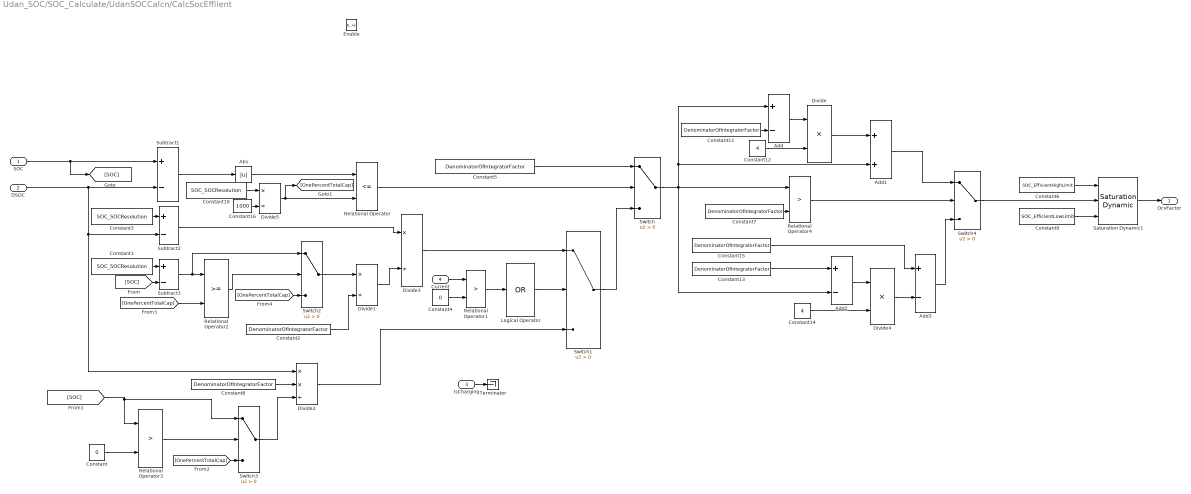
== system Udan_SOC/SOC_Calculate/UdanSOCCalcn/CalcSocEffiient ==
  SOC : Inport
  DSOC : Inport  Port=2
  IsCharging : Inport  Port=3
  Current : Inport  Port=4
  Enable : EnablePort
  Abs : Abs
  Add : Sum  Inputs=+-  AccumDataTypeStr=int32  OutDataTypeStr=int32
  Add1 : Sum  AccumDataTypeStr=int32  OutDataTypeStr=int32
  Add2 : Sum  Inputs=+-  AccumDataTypeStr=int32  OutDataTypeStr=int32
  Add3 : Sum  Inputs=+-  AccumDataTypeStr=int32  OutDataTypeStr=int32
  Constant : Constant  Value=0  OutDataTypeStr=uint8
  Constant1 : Constant  Value=SOC_SOCResolution
  Constant10 : Constant  Value=SOC_SOCResolution
  Constant{7,11,13,15} (4 alike) : Constant  Value=DenominatorOfIntegratorFactor  OutDataTypeStr=uint8
  Constant12 : Constant  Value=4  OutDataTypeStr=uint8
  Constant14 : Constant  Value=4  OutDataTypeStr=uint8
  Constant16 : Constant  Value=1000  OutDataTypeStr=uint16
  Constant2 : Constant  Value=DenominatorOfIntegratorFactor  OutDataTypeStr=uint16
  Constant3 : Constant  Value=SOC_SOCResolution
  Constant4 : Constant  Value=0  OutDataTypeStr=uint16
  Constant5 : Constant  Value=DenominatorOfIntegratorFactor  OutDataTypeStr=uint16
  Constant6 : Constant  Value=SOC_EfficientHighLimit  OutDataTypeStr=uint16
  Constant8 : Constant  Value=DenominatorOfIntegratorFactor  OutDataTypeStr=uint16
  Constant9 : Constant  Value=SOC_EfficientLowLimit  OutDataTypeStr=uint16
  Divide : Product  Inputs=**  OutDataTypeStr=int32
  Divide1 : Product  Inputs=*/  OutDataTypeStr=int32
  Divide2 : Product  Inputs=**/  OutDataTypeStr=int32
  Divide3 : Product  Inputs=*/  OutDataTypeStr=int32
  Divide4 : Product  Inputs=**  OutDataTypeStr=int32
  Divide5 : Product  Inputs=*/  OutDataTypeStr=uint32
  Logical Operator : Logic  Operator=OR  Inputs=1  AllPortsSameDT=off  OutDataTypeStr=boolean
  Relational Operator : RelationalOperator  Operator=<=  OutDataTypeStr=boolean  RndMeth=Nearest
  Relational Operator1 : RelationalOperator  Operator=>  OutDataTypeStr=boolean  RndMeth=Nearest
  Relational Operator2 : RelationalOperator  OutDataTypeStr=boolean  RndMeth=Simplest
  Relational Operator3 : RelationalOperator  Operator=>  OutDataTypeStr=boolean  RndMeth=Simplest
  Relational Operator4 : RelationalOperator  Operator=>  OutDataTypeStr=boolean  RndMeth=Simplest
  Saturation Dynamic1 : simulink/Discontinuities/Saturation Dynamic  OutMin=[]  OutMax=[]  OutDataTypeStr=uint16  OutputDataTypeScalingMode=uint16  OutDataType=fixdt(1, 16)  OutScaling=2^-10  DoSatur=off
  Subtract1 : Sum  Inputs=+-  OutDataTypeStr=int32
  Subtract2 : Sum  Inputs=+-  OutDataTypeStr=int32
  Subtract3 : Sum  Inputs=+-  OutDataTypeStr=int32
  Switch : Switch  Criteria=u2 > Threshold  OutDataTypeStr=uint16  RndMeth=Round
  Switch1 : Switch  Criteria=u2 > Threshold  OutDataTypeStr=uint16  RndMeth=Round
  Switch2 : Switch  Criteria=u2 > Threshold
  Switch3 : Switch  Criteria=u2 > Threshold
  Switch4 : Switch  Criteria=u2 > Threshold  OutDataTypeStr=int32
  Terminator : Terminator
  OcvFactor : Outport
  wires:
  Constant16/1 -> Divide5/2
  Divide5/1 -> Relational Operator/2, [OnePercentTotalCap]
  Constant10/1 -> Divide5/1
  Divide1/1 -> Divide3/2
  Constant2/1 -> Divide1/2
  [OnePercentTotalCap] -> Switch2/3
  Relational Operator2/1 -> Switch2/2
  [OnePercentTotalCap] -> Relational Operator2/2
  Subtract3/1 -> Switch2/1, Relational Operator2/1
  Constant1/1 -> Subtract3/1
  [SOC] -> Subtract3/2
  Relational Operator1/1 -> Logical Operator/1
  Logical Operator/1 -> Switch1/2
  Constant4/1 -> Relational Operator1/2
  Current/1 -> Relational Operator1/1
  Divide3/1 -> Switch1/1
  IsCharging/1 -> Terminator/1
  SOC/1 -> Subtract1/1, [SOC]
  Subtract2/1 -> Divide3/1
  Constant3/1 -> Subtract2/1
  DSOC/1 -> Subtract1/2, Divide2/1, Subtract2/2
  Switch2/1 -> Divide1/1
  Switch1/1 -> Switch/3
  Subtract1/1 -> Abs/1
  Relational Operator/1 -> Switch/2
  Abs/1 -> Relational Operator/1
  Constant5/1 -> Switch/1
  Saturation Dynamic1/1 -> OcvFactor/1
  Constant/1 -> Relational Operator3/2
  [SOC] -> Relational Operator3/1, Switch3/1
  Constant8/1 -> Divide2/2
  Divide2/1 -> Switch1/3
  Relational Operator3/1 -> Switch3/2
  Switch3/1 -> Divide2/3
  [OnePercentTotalCap] -> Switch3/3
  Switch4/1 -> Saturation Dynamic1/2
  Constant9/1 -> Saturation Dynamic1/3
  Constant6/1 -> Saturation Dynamic1/1
  Switch/1 -> Add2/2, Add/1, Add1/2, Relational Operator4/1
  Constant7/1 -> Relational Operator4/2
  Relational Operator4/1 -> Switch4/2
  Constant11/1 -> Add/2
  Add/1 -> Divide/1
  Constant12/1 -> Divide/2
  Divide/1 -> Add1/1
  Add1/1 -> Switch4/1
  Constant13/1 -> Add2/1
  Add2/1 -> Divide4/1
  Constant14/1 -> Divide4/2
  Divide4/1 -> Add3/2
  Add3/1 -> Switch4/3
  Constant15/1 -> Add3/1
